simulink model "servo_controller_motor"  (R2024b)
settings: Solver=VariableStepAuto  StartTime=0.0  StopTime=30  RelTol=1e-3
undefined symbols (not defined in the file): b, J, Kd, ke, Ki, Kp, kt, L, Nf, R, Tsample
settings Model: Creator=omari  LastModifiedBy=omari

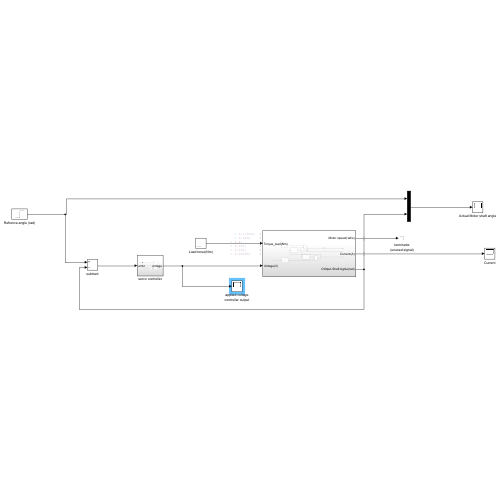
[thumbnail: Simulink's stored preview of the top-level diagram]
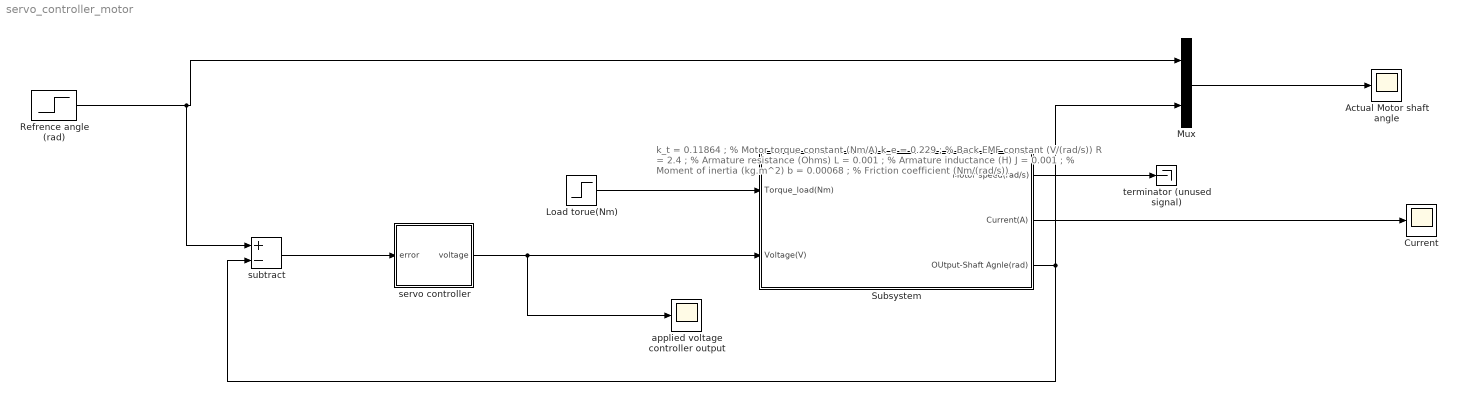
== system servo_controller_motor ==
  note: k_t = 0.11864 ; % Motor torque constant (Nm/A)
      | k_e = 0.229 ; % Back EMF constant (V/(rad/s))
      | R = 2.4 ; % Armature resistance (Ohms)
      | L = 0.001 ; % Armature inductance (H)
      | J = 0.001 ; % Moment of inertia (kg.m^2)
      | b = 0.00068 ; % Friction coefficient (Nm/(rad/s))
  Actual Motor shaft angle : Scope
  Current : Scope
  Load torue(Nm) : Step  After=0  SampleTime=Tsample
  Mux : Mux  Inputs=2
  Refrence angle (rad) : Step  After=pi/3  SampleTime=Tsample
  Subsystem : Subsystem
  applied voltage controller output : Scope
  servo controller : Subsystem
  subtract : Sum  Inputs=+-
  terminator (unused signal) : Terminator
  wires:
  Subsystem/1(Motor speed(rad/s)) -> terminator (unused signal)/1
  servo controller/1(voltage) -> applied voltage controller output/1, Subsystem/2(Voltage(V))
  Load torue(Nm)/1 -> Subsystem/1(Torque_load(Nm))
  Refrence angle (rad)/1 -> subtract/1, Mux/1
  subtract/1 -> servo controller/1(error)
  Subsystem/2(Current(A)) -> Current/1
  Subsystem/3(OUtput-Shaft Agnle(rad)) -> subtract/2, Mux/2
  Mux/1 -> Actual Motor shaft angle/1

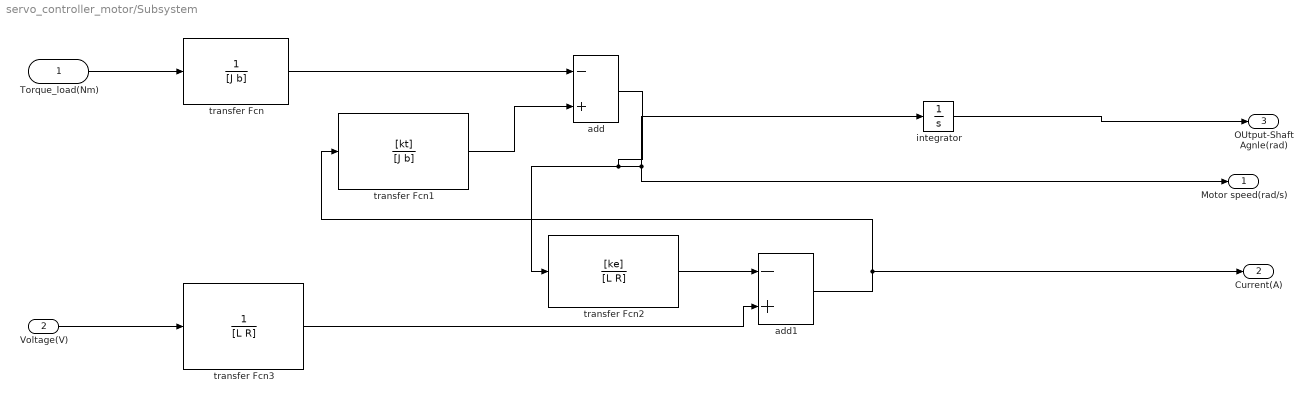
== system servo_controller_motor/Subsystem ==
  Torque_load(Nm) : Inport
  Voltage(V) : Inport  Port=2
  add : Sum  Inputs=-+
  add1 : Sum  Inputs=-+
  integrator : Integrator
  transfer Fcn : TransferFcn  Denominator=[J b]
  transfer Fcn1 : TransferFcn  Numerator=[kt]  Denominator=[J b]
  transfer Fcn2 : TransferFcn  Numerator=[ke]  Denominator=[L R]
  transfer Fcn3 : TransferFcn  Denominator=[L R]
  Motor speed(rad/s) : Outport
  Current(A) : Outport  Port=2
  OUtput-Shaft Agnle(rad) : Outport  Port=3
  wires:
  add/1 -> transfer Fcn2/1, Motor speed(rad/s)/1, integrator/1
  add1/1 -> Current(A)/1, transfer Fcn1/1
  Torque_load(Nm)/1 -> transfer Fcn/1
  transfer Fcn3/1 -> add1/2
  transfer Fcn2/1 -> add1/1
  Voltage(V)/1 -> transfer Fcn3/1
  transfer Fcn/1 -> add/1
  transfer Fcn1/1 -> add/2
  integrator/1 -> OUtput-Shaft Agnle(rad)/1

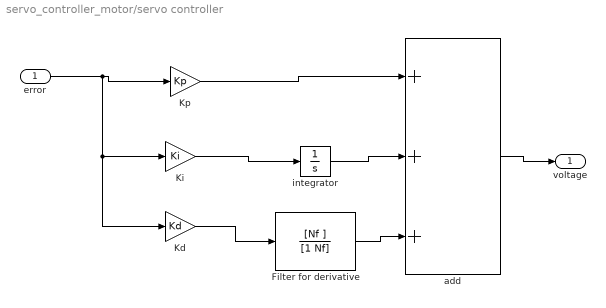
== system servo_controller_motor/servo controller ==
  error : Inport
  Filter for derivative : TransferFcn  Numerator=[Nf ]  Denominator=[1 Nf]
  Kd : Gain  Gain=Kd
  Ki : Gain  Gain=Ki
  Kp : Gain  Gain=Kp
  add : Sum  Inputs=+++
  integrator : Integrator
  voltage : Outport
  wires:
  error/1 -> Kd/1, Ki/1, Kp/1
  Filter for derivative/1 -> add/3
  Kd/1 -> Filter for derivative/1
  Kp/1 -> add/1
  integrator/1 -> add/2
  Ki/1 -> integrator/1
  add/1 -> voltage/1
